simulink model "aspa_2w_towed__modular"  (R2016a)
settings: Solver=VariableStepAuto  StartTime=0.0  StopTime=100  RelTol=1e-3
undefined symbols (not defined in the file): b1, b2, I, k1, k2, k3, k4, LF, LR, M_sb, M_UsbF, M_UsbR
settings Model: Creator=mm395  LastModifiedBy=mm395
settings GRTTargetCC: GeneratePreprocessorConditionals=Use local settings

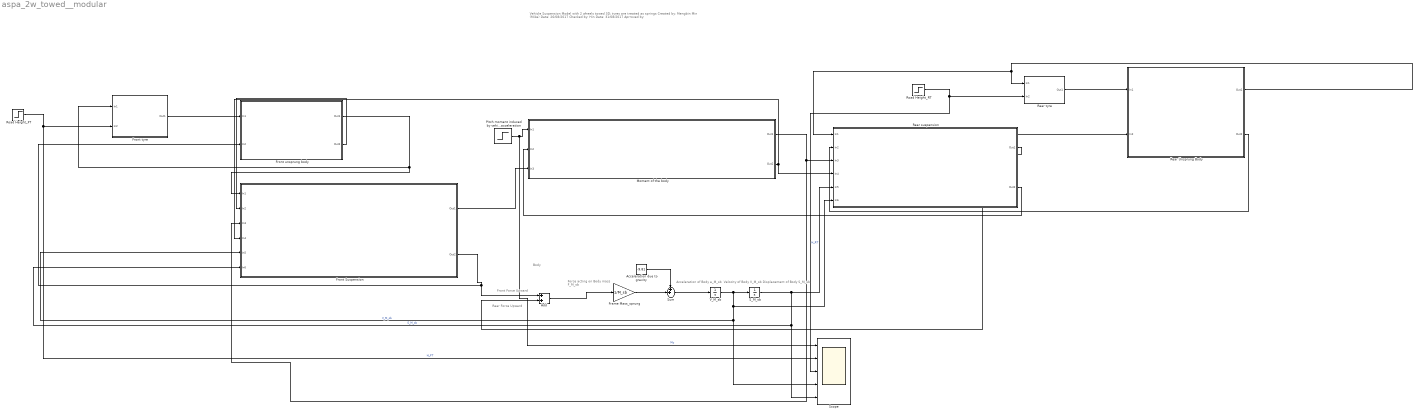
== system aspa_2w_towed__modular ==
  note: Rear Force Upward
  note: Front Force Upward
  note: Body
  note: Acceleration of Body
      | a_M_sb
  note: Force acting on Body mass
      | F_M_sb
  note: Velocity of Body
      | V_M_sb
  note: Displacement of Body
      | S_M_sb
  note: Vehicle Suspension Model with 2 wheels towed
      | 3D; tyres are treated as springs
      | Created by: Mengbin Min (Mike) Date: 26/08/2017
      | Checked by: Hin Date: 31/08/2017
      | Aprroved by:
  Acceleration due to gravity : Constant  Value=-9.81
  Add : Sum
  Frame Mass_sprung : Gain  Gain=1/M_sb
  Front Suspension : Subsystem
  Front tyre : Subsystem
  Front unsprung body : Subsystem
  Moment of the body : Subsystem
  Pitch moment induced by vehicle acceleration : Step  After=100  SampleTime=0
  Rear Unsprung Body : Subsystem
  Rear suspension : Subsystem
  Rear tyre : Subsystem
  Road Height_FT : Step  Time=2  After=0.05  SampleTime=0
  Road Height_RT : Step  Time=4  After=0.05  SampleTime=0
  S_M_sb : Integrator
  Scope : Scope  NumInputPorts=5
  Sum : Sum  Inputs=++|
  V_M_sb : Integrator
  wires:
  Add/1 -> Frame Mass_sprung/1
  Frame Mass_sprung/1 -> Sum/2
  Acceleration due to gravity/1 -> Sum/1
  V_M_sb/1 -> Rear suspension/6(In6), Front Suspension/5(In5), Scope/4, S_M_sb/1  "V_M_sb"
  S_M_sb/1 -> Rear suspension/5(In5), Front Suspension/6(In6), Scope/5  "S_M_sb"
  Sum/1 -> V_M_sb/1
  Pitch moment induced by vehicle acceleration/1 -> Moment of the body/1(In1), Scope/1  "My"
  Road Height_RT/1 -> Rear tyre/2(In2), Scope/3  "H_RT"
  Road Height_FT/1 -> Front tyre/2(In2), Scope/2  "H_FT"
  Rear Unsprung Body/1(Out1) -> Rear tyre/1(In1), Rear suspension/1(In1)
  Rear suspension/1(Out1) -> Rear Unsprung Body/2(In2), Add/2
  Rear Unsprung Body/2(Out2) -> Rear suspension/2(In2)
  Rear tyre/1(Out1) -> Rear Unsprung Body/1(In1)
  Moment of the body/2(Out2) -> Front Suspension/4(In4), Rear suspension/4(In4)
  Moment of the body/1(Out1) -> Front Suspension/3(In3), Rear suspension/3(In3)
  Rear suspension/2(Out2) -> Moment of the body/2(In2)
  Front unsprung body/1(Out1) -> Front Suspension/1(In1), Front tyre/1(In1)
  Front tyre/1(Out1) -> Front unsprung body/1(In1)
  Front Suspension/2(Out2) -> Front unsprung body/2(In2), Add/1
  Front unsprung body/2(Out2) -> Front Suspension/2(In2)
  Front Suspension/1(Out1) -> Moment of the body/3(In3)

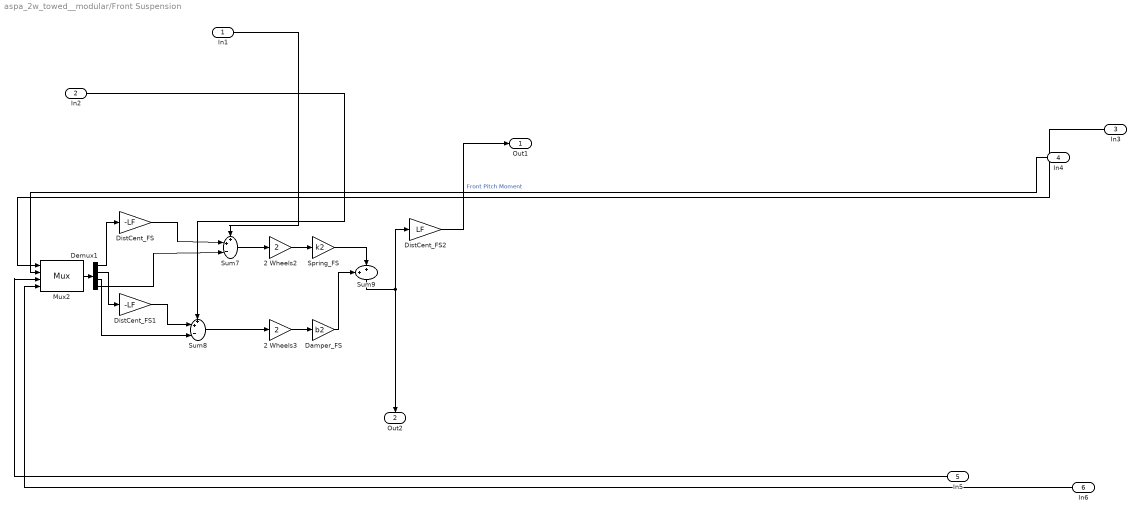
== system aspa_2w_towed__modular/Front Suspension ==
  In1 : Inport
  In2 : Inport  Port=2
  In3 : Inport  Port=3
  In4 : Inport  Port=4
  In5 : Inport  Port=5
  In6 : Inport  Port=6
  2 Wheels2 : Gain  Gain=2
  2 Wheels3 : Gain  Gain=2
  Damper_FS : Gain  Gain=b2
  Demux1 : Demux
  DistCent_FS : Gain  Gain=-LF
  DistCent_FS1 : Gain  Gain=-LF
  DistCent_FS2 : Gain  Gain=LF
  Mux2 : Mux
      settings: DisplayOption=signals
  Spring_FS : Gain  Gain=k2
  Sum7 : Sum  Inputs=++-|
  Sum8 : Sum  Inputs=++-|
  Sum9 : Sum  Inputs=++|
  Out1 : Outport
  Out2 : Outport  Port=2
  wires:
  In2/1 -> Sum8/1
  In5/1 -> Mux2/3
  In3/1 -> Mux2/1
  In6/1 -> Mux2/4
  In4/1 -> Mux2/2
  In1/1 -> Sum7/1
  DistCent_FS2/1 -> Out1/1  "Front Pitch Moment"
  Mux2/1 -> Demux1/1
  Spring_FS/1 -> Sum9/2
  Damper_FS/1 -> Sum9/1
  Demux1/1 -> DistCent_FS/1
  Demux1/3 -> Sum8/3
  Demux1/4 -> Sum7/3
  DistCent_FS/1 -> Sum7/2
  Sum8/1 -> 2 Wheels3/1
  Demux1/2 -> DistCent_FS1/1
  DistCent_FS1/1 -> Sum8/2
  Sum7/1 -> 2 Wheels2/1
  2 Wheels2/1 -> Spring_FS/1
  2 Wheels3/1 -> Damper_FS/1
  Sum9/1 -> Out2/1, DistCent_FS2/1

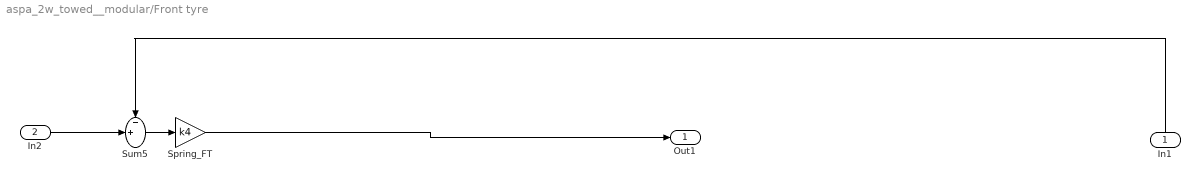
== system aspa_2w_towed__modular/Front tyre ==
  In1 : Inport
  In2 : Inport  Port=2
  Spring_FT : Gain  Gain=k4
  Sum5 : Sum  Inputs=-+|
  Out1 : Outport
  wires:
  In1/1 -> Sum5/1
  Spring_FT/1 -> Out1/1
  In2/1 -> Sum5/2
  Sum5/1 -> Spring_FT/1

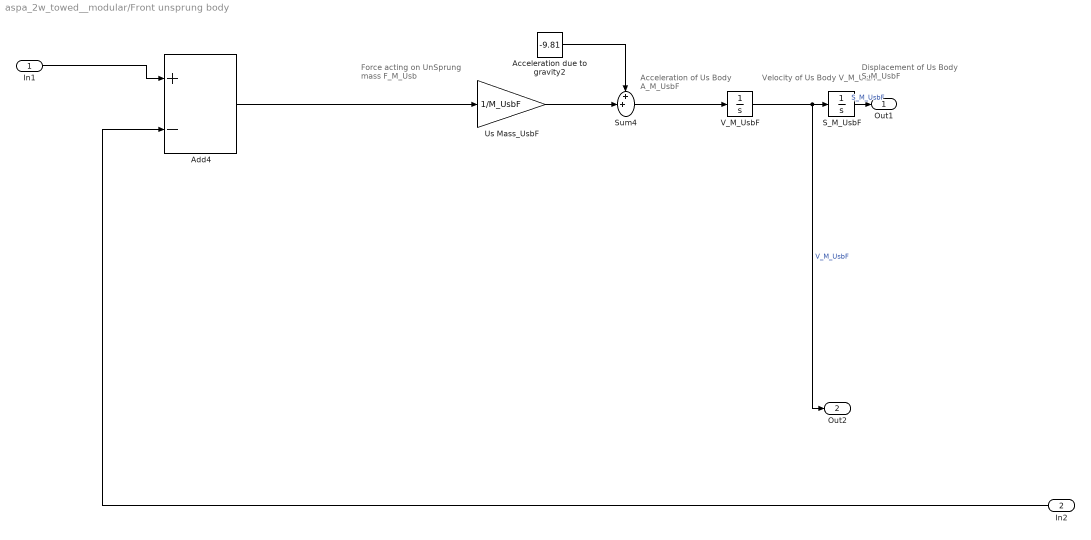
== system aspa_2w_towed__modular/Front unsprung body ==
  note: Acceleration of Us Body
      | A_M_UsbF
  note: Force acting on UnSprung mass
      | F_M_Usb
  note: Velocity of Us Body
      | V_M_UsbF
  note: Displacement of Us Body
      | S_M_UsbF
  In1 : Inport
  In2 : Inport  Port=2
  Acceleration due to gravity2 : Constant  Value=-9.81
  Add4 : Sum  Inputs=+-
  S_M_UsbF : Integrator
  Sum4 : Sum  Inputs=++|
  Us Mass_UsbF : Gain  Gain=1/M_UsbF
  V_M_UsbF : Integrator
  Out1 : Outport
  Out2 : Outport  Port=2
  wires:
  In2/1 -> Add4/2
  Acceleration due to gravity2/1 -> Sum4/1
  V_M_UsbF/1 -> Out2/1, S_M_UsbF/1  "V_M_UsbF"
  Add4/1 -> Us Mass_UsbF/1
  Us Mass_UsbF/1 -> Sum4/2
  S_M_UsbF/1 -> Out1/1  "S_M_UsbF"
  Sum4/1 -> V_M_UsbF/1
  In1/1 -> Add4/1

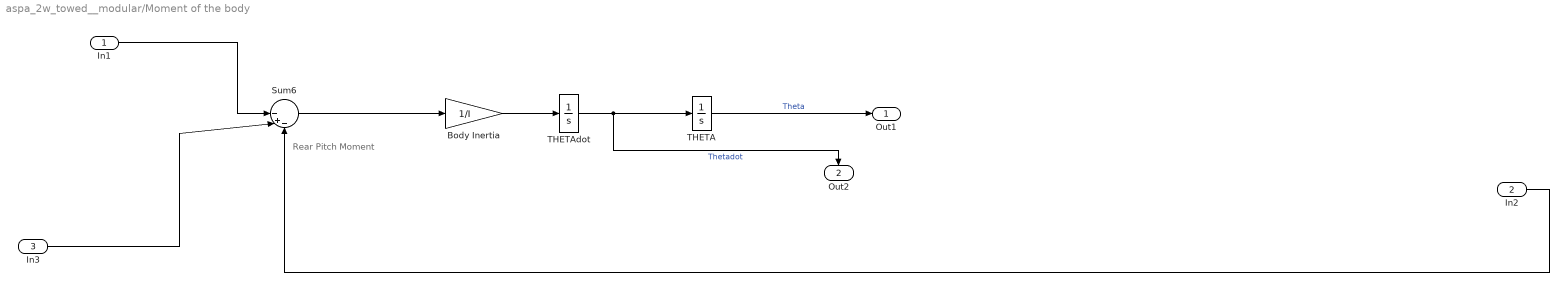
== system aspa_2w_towed__modular/Moment of the body ==
  note: Rear Pitch Moment
  In1 : Inport
  In2 : Inport  Port=2
  In3 : Inport  Port=3
  Body Inertia : Gain  Gain=1/I  SaturateOnIntegerOverflow=on  OutDataTypeStr=Inherit: Same as input  ParamDataTypeStr=Inherit: Same as input
  Sum6 : Sum  Inputs=||-+-  SaturateOnIntegerOverflow=on  InputSameDT=on  OutDataTypeStr=Inherit: Same as first input
  THETA : Integrator  InitialCondition=-8.7e-20
  THETAdot : Integrator  InitialCondition=8.04e-28
  Out1 : Outport
  Out2 : Outport  Port=2
  wires:
  In2/1 -> Sum6/3
  In1/1 -> Sum6/1
  THETAdot/1 -> Out2/1, THETA/1  "Thetadot"
  THETA/1 -> Out1/1  "Theta"
  In3/1 -> Sum6/2
  Body Inertia/1 -> THETAdot/1
  Sum6/1 -> Body Inertia/1

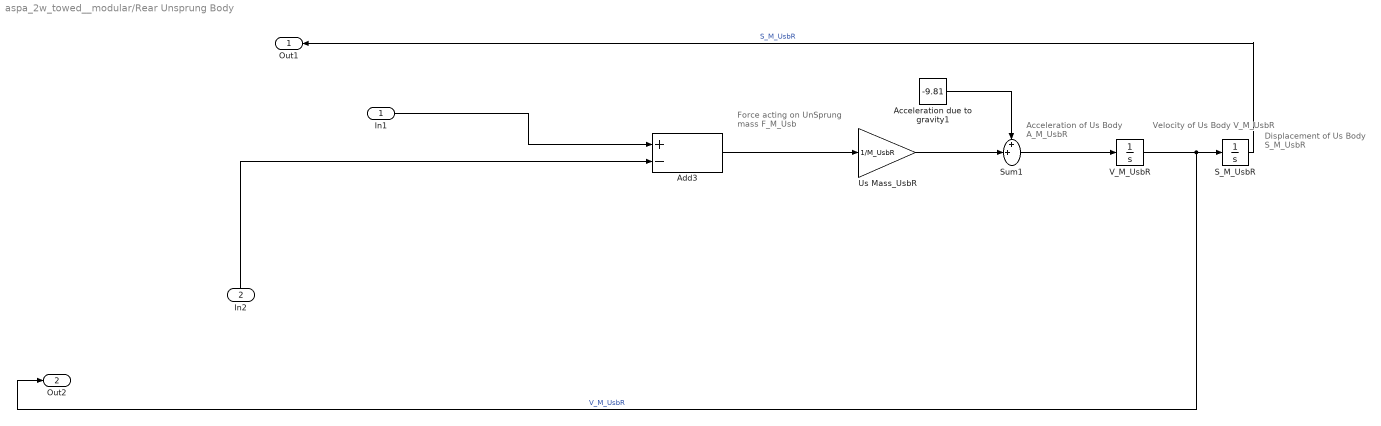
== system aspa_2w_towed__modular/Rear Unsprung Body ==
  note: Acceleration of Us Body
      | A_M_UsbR
  note: Force acting on UnSprung mass
      | F_M_Usb
  note: Velocity of Us Body
      | V_M_UsbR
  note: Displacement of Us Body
      | S_M_UsbR
  In1 : Inport
  In2 : Inport  Port=2
  Acceleration due to gravity1 : Constant  Value=-9.81
  Add3 : Sum  Inputs=+-
  S_M_UsbR : Integrator
  Sum1 : Sum  Inputs=++|
  Us Mass_UsbR : Gain  Gain=1/M_UsbR
  V_M_UsbR : Integrator
  Out1 : Outport
  Out2 : Outport  Port=2
  wires:
  In2/1 -> Add3/2
  V_M_UsbR/1 -> Out2/1, S_M_UsbR/1  "V_M_UsbR"
  Sum1/1 -> V_M_UsbR/1
  S_M_UsbR/1 -> Out1/1  "S_M_UsbR"
  Acceleration due to gravity1/1 -> Sum1/1
  Us Mass_UsbR/1 -> Sum1/2
  In1/1 -> Add3/1
  Add3/1 -> Us Mass_UsbR/1

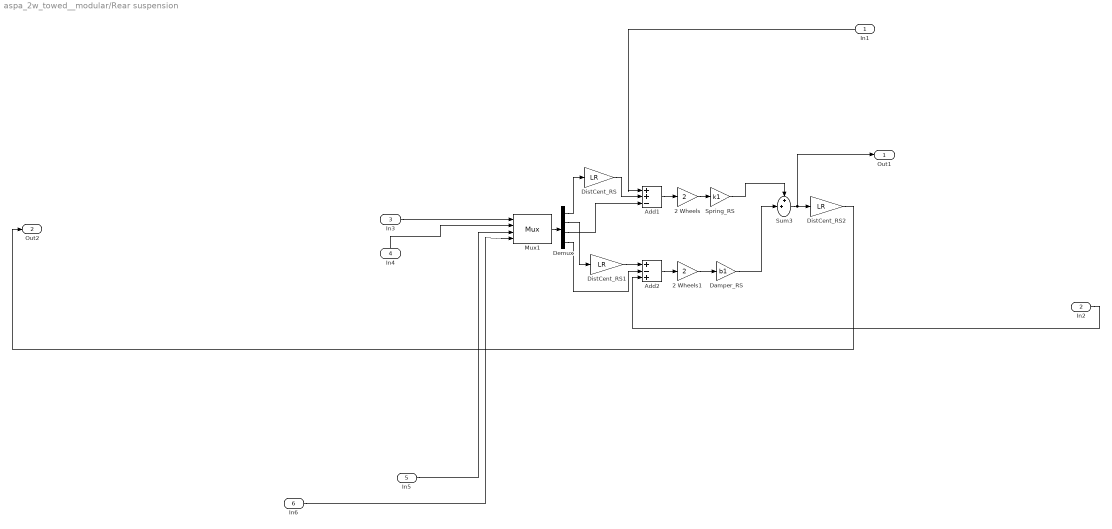
== system aspa_2w_towed__modular/Rear suspension ==
  In1 : Inport
  In2 : Inport  Port=2
  In3 : Inport  Port=3
  In4 : Inport  Port=4
  In5 : Inport  Port=5
  In6 : Inport  Port=6
  2 Wheels : Gain  Gain=2
  2 Wheels1 : Gain  Gain=2
  Add1 : Sum  Inputs=++-
  Add2 : Sum  Inputs=+-+
  Damper_RS : Gain  Gain=b1
  Demux : Demux
  DistCent_RS : Gain  Gain=LR
  DistCent_RS1 : Gain  Gain=LR
  DistCent_RS2 : Gain  Gain=LR
  Mux1 : Mux
      settings: DisplayOption=signals
  "Spring_RS " : Gain  Gain=k1
  Sum3 : Sum  Inputs=++|
  Out1 : Outport
  Out2 : Outport  Port=2
  wires:
  In2/1 -> Add2/3
  In4/1 -> Mux1/2
  In6/1 -> Mux1/4
  Sum3/1 -> DistCent_RS2/1, Out1/1
  In5/1 -> Mux1/3
  In3/1 -> Mux1/1
  In1/1 -> Add1/1
  Demux/1 -> DistCent_RS/1
  Demux/3 -> Add1/3
  Damper_RS/1 -> Sum3/2
  Demux/2 -> DistCent_RS1/1
  DistCent_RS1/1 -> Add2/1
  "Spring_RS "/1 -> Sum3/1
  DistCent_RS2/1 -> Out2/1
  Add2/1 -> 2 Wheels1/1
  2 Wheels1/1 -> Damper_RS/1
  2 Wheels/1 -> "Spring_RS "/1
  Add1/1 -> 2 Wheels/1
  Demux/4 -> Add2/2
  Mux1/1 -> Demux/1
  DistCent_RS/1 -> Add1/2

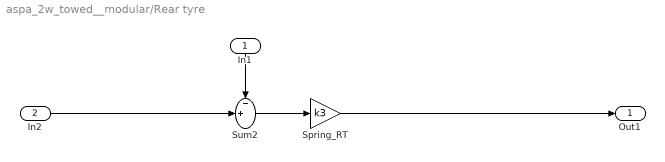
== system aspa_2w_towed__modular/Rear tyre ==
  In1 : Inport
  In2 : Inport  Port=2
  Spring_RT : Gain  Gain=k3
  Sum2 : Sum  Inputs=-+|
  Out1 : Outport
  wires:
  Spring_RT/1 -> Out1/1
  In2/1 -> Sum2/2
  In1/1 -> Sum2/1
  Sum2/1 -> Spring_RT/1
